simulink subsystem "robot_model_bus_7dof_ref_subsys"  (R2022b)
settings: Solver=VariableStepAuto  StartTime=0.0  StopTime=10.0  RelTol=1e-3
undefined symbols (not defined in the file): param_global
libraries: simulink x1
settings Model: Creator=emu  LastModifiedBy=emu
settings OptimizationCC: ReuseModelBlockBuffer=on

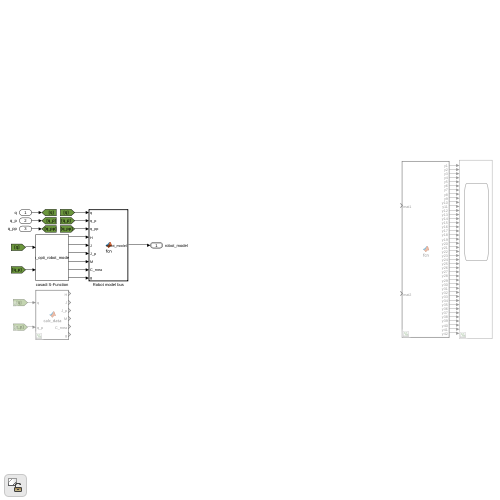
[thumbnail: Simulink's stored preview of the top-level diagram]
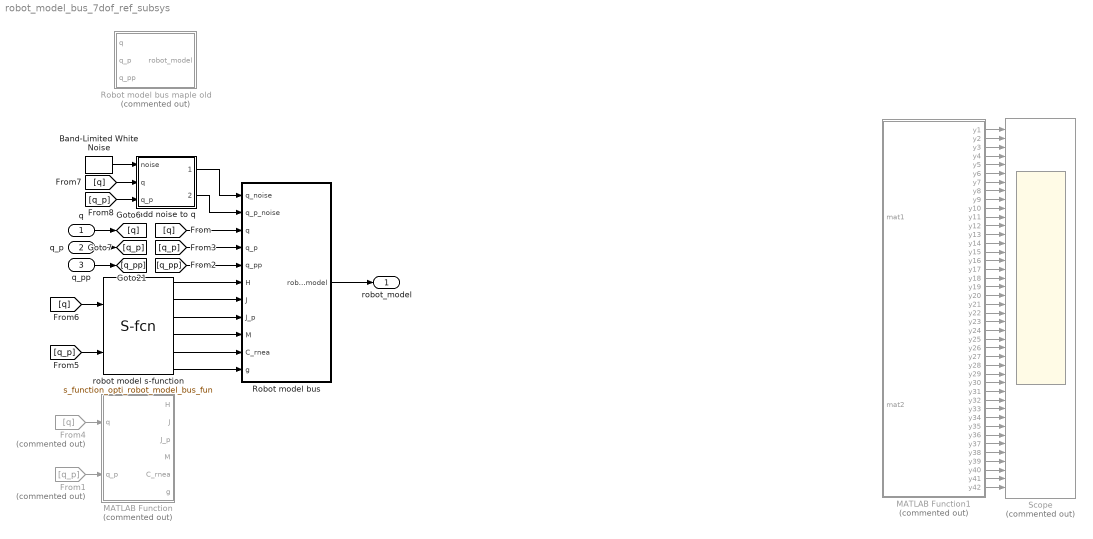
== system robot_model_bus_7dof_ref_subsys ==
  q : Inport
  q_p : Inport  Port=2
  q_pp : Inport  Port=3
  Band-Limited White Noise : simulink/Sources/Band-Limited White Noise  Cov=[1e-6]  Ts=param_global.Ta  seed=[23341]
  From1 : From  Commented=on  GotoTag=q_p
  From4 : From  Commented=on  GotoTag=q
  MATLAB Function : MATLAB Function  Commented=on  TreatAsAtomicUnit=on
  MATLAB Function1 : MATLAB Function  Commented=on  TreatAsAtomicUnit=on
  Robot model bus : MATLAB Function  TreatAsAtomicUnit=on
  Robot model bus maple old : MATLAB Function  Commented=on  TreatAsAtomicUnit=on
  Scope : Scope  Commented=on  NumInputPorts=42
  add noise to q : MATLAB Function  TreatAsAtomicUnit=on
  robot model s-function : S-Function  FunctionName=s_function_opti_robot_model_bus_fun  SFunctionModules='robot_model_bus_fun'  SFunctionDeploymentMode=off  EnableBusSupport=off
  robot_model : Outport  OutDataTypeStr=Bus: robot_model
  wires:
  Robot model bus/1(robot_model) -> robot_model/1
  robot model s-function/3 -> Robot model bus/8(J_p)
  robot model s-function/4 -> Robot model bus/9(M)
  robot model s-function/6 -> Robot model bus/11(g)
  q_pp/1 -> [q_pp]
  q_p/1 -> [q_p]
  q/1 -> [q]
  [q] -> Robot model bus/3(q)
  [q_p] -> Robot model bus/4(q_p)
  [q_pp] -> Robot model bus/5(q_pp)
  From4/1 -> MATLAB Function/1(q)
  From1/1 -> MATLAB Function/2(q_p)
  [q_p] -> robot model s-function/2
  [q] -> robot model s-function/1
  robot model s-function/5 -> Robot model bus/10(C_rnea)
  robot model s-function/1 -> Robot model bus/6(H)
  robot model s-function/2 -> Robot model bus/7(J)
  MATLAB Function1/1(y1) -> Scope/1
  MATLAB Function1/2(y2) -> Scope/2
  MATLAB Function1/3(y3) -> Scope/3
  MATLAB Function1/4(y4) -> Scope/4
  MATLAB Function1/5(y5) -> Scope/5
  MATLAB Function1/6(y6) -> Scope/6
  MATLAB Function1/7(y7) -> Scope/7
  MATLAB Function1/8(y8) -> Scope/8
  MATLAB Function1/9(y9) -> Scope/9
  MATLAB Function1/10(y10) -> Scope/10
  MATLAB Function1/11(y11) -> Scope/11
  MATLAB Function1/12(y12) -> Scope/12
  MATLAB Function1/13(y13) -> Scope/13
  MATLAB Function1/14(y14) -> Scope/14
  MATLAB Function1/15(y15) -> Scope/15
  MATLAB Function1/16(y16) -> Scope/16
  MATLAB Function1/17(y17) -> Scope/17
  MATLAB Function1/18(y18) -> Scope/18
  MATLAB Function1/19(y19) -> Scope/19
  MATLAB Function1/20(y20) -> Scope/20
  MATLAB Function1/21(y21) -> Scope/21
  MATLAB Function1/22(y22) -> Scope/22
  MATLAB Function1/23(y23) -> Scope/23
  MATLAB Function1/24(y24) -> Scope/24
  MATLAB Function1/25(y25) -> Scope/25
  MATLAB Function1/26(y26) -> Scope/26
  MATLAB Function1/27(y27) -> Scope/27
  MATLAB Function1/28(y28) -> Scope/28
  MATLAB Function1/29(y29) -> Scope/29
  MATLAB Function1/30(y30) -> Scope/30
  MATLAB Function1/31(y31) -> Scope/31
  MATLAB Function1/32(y32) -> Scope/32
  MATLAB Function1/33(y33) -> Scope/33
  MATLAB Function1/34(y34) -> Scope/34
  MATLAB Function1/35(y35) -> Scope/35
  MATLAB Function1/36(y36) -> Scope/36
  MATLAB Function1/37(y37) -> Scope/37
  MATLAB Function1/38(y38) -> Scope/38
  MATLAB Function1/39(y39) -> Scope/39
  MATLAB Function1/40(y40) -> Scope/40
  MATLAB Function1/41(y41) -> Scope/41
  MATLAB Function1/42(y42) -> Scope/42
  Band-Limited White Noise/1 -> add noise to q/1(noise)
  [q] -> add noise to q/2(q)
  [q_p] -> add noise to q/3(q_p)
  add noise to q/2(q_p_noise) -> Robot model bus/2(q_p_noise)
  add noise to q/1(q_noise) -> Robot model bus/1(q_noise)

== matlab function robot_model_bus_7dof_ref_subsys/Robot model bus maple old ==
  settings: updateMethod=DISCRETE  sampleTime=param_global.Ta
  data: q input; q_p input; q_pp input; robot_model output Bus: robot_model; param_robot parameter
function robot_model = fcn(q, q_p, q_pp, param_robot)
% Parameters
robot_model=struct();
robot_model.q=q;                    % generalized coordinates
robot_model.q_p=q_p;                % time derivative of generalized coordinates
robot_model.q_pp=q_pp;
robot_model.H=hom_transform_endeffector(q, param_robot);            % homogenous transformation to end-effector
robot_model.J=geo_jacobian_endeffector(q,param_robot);              % geometric jacobian to end-effector
robot_model.J_p=geo_jacobian_endeffector_p(q, q_p,param_robot);     % time derivative of geometric jacobian to end-effector
robot_model.M=inertia_matrix(q,param_robot);                        % inertia matrix
robot_model.C=coriolis_matrix(q, q_p,param_robot);                  % coriolis matrix
robot_model.g=gravitational_forces(q,param_robot);                  % gravitational forces
end

== matlab function robot_model_bus_7dof_ref_subsys/add noise to q ==
  data: noise input; q_noise output; q input; q_p input; q_p_noise output; param_global parameter
function [q_noise, q_p_noise] = fcn(noise, q, q_p, param_global)

q_noise = q + noise;
q_p_noise = q_p + param_global.Ta*noise;

== matlab function robot_model_bus_7dof_ref_subsys/Robot model bus ==
  settings: updateMethod=DISCRETE  sampleTime=param_global.Ta
  data: q_noise input; q_p_noise input; q input; q_p input; q_pp input; H input; J input; J_p input; M input; C_rnea input; g input; robot_model output Bus: robot_model
function robot_model = fcn(q_noise, q_p_noise, q, q_p, q_pp, H, J, J_p, M, C_rnea, g)
% Parameters
robot_model=struct();
robot_model.q_noise = q_noise;
robot_model.q_p_noise = q_p_noise;
robot_model.q=q;                    % generalized coordinates
robot_model.q_p=q_p;                % time derivative of generalized coordinates
robot_model.q_pp=q_pp;
robot_model.H=H;
robot_model.J=J;
robot_model.J_p=J_p;
robot_model.M=M;
robot_model.C_rnea=C_rnea; % C_rnea(q, q_p) = C(q, q_p)q_p + g(q) = n(q, q_p)
robot_model.g=g;
end

== matlab function robot_model_bus_7dof_ref_subsys/MATLAB Function ==
  data: q input; H output; q_p input; J output; J_p output; M output; C_rnea output; g output; param_robot parameter
function [H, J, J_p, M, C_rnea, g] = calc_data(q, q_p, param_robot)

H=hom_transform_endeffector(q, param_robot);            % homogenous transformation to end-effector
J=geo_jacobian_endeffector(q,param_robot);              % geometric jacobian to end-effector
J_p=geo_jacobian_endeffector_p(q, q_p,param_robot);     % time derivative of geometric jacobian to end-effector
M=inertia_matrix(q,param_robot);                        % inertia matrix
g=gravitational_forces(q,param_robot);                  % gravitational forces
C_rnea=coriolis_matrix(q, q_p,param_robot)*q_p + g;     % coriolis matrix

== matlab function robot_model_bus_7dof_ref_subsys/MATLAB Function1 ==
  data: mat1 input; y1 output Bus: test_bus; mat2 input; y2 output Bus: test_bus; y3 output Bus: test_bus; y4 output Bus: test_bus; y5 output Bus: test_bus; y6 output Bus: test_bus; y7 output Bus: test_bus; y8 output Bus: test_bus; y9 output Bus: test_bus; y10 output Bus: test_bus; y11 output Bus: test_bus; y12 output Bus: test_bus; y13 output Bus: test_bus; y14 output Bus: test_bus; y15 output Bus: test_bus; y16 output Bus: test_bus; y17 output Bus: test_bus; y18 output Bus: test_bus; y19 output Bus: test_bus; y20 output Bus: test_bus; y21 output Bus: test_bus; y22 output Bus: test_bus; y23 output Bus: test_bus; y24 output Bus: test_bus; y25 output Bus: test_bus; y26 output Bus: test_bus; y27 output Bus: test_bus; y28 output Bus: test_bus; y29 output Bus: test_bus; y30 output Bus: test_bus; y31 output Bus: test_bus; y32 output Bus: test_bus; y33 output Bus: test_bus; y34 output Bus: test_bus; y35 output Bus: test_bus; y36 output Bus: test_bus; y37 output Bus: test_bus; y38 output Bus: test_bus; y39 output Bus: test_bus; y40 output Bus: test_bus; y41 output Bus: test_bus; y42 output Bus: test_bus; init_bus_param parameter
function [y1, y2, y3, y4, y5, y6, y7, y8, y9, y10, y11, y12, y13, y14, y15, y16, y17, y18, y19, y20, y21, y22, y23, y24, y25, y26, y27, y28, y29, y30, y31, y32, y33, y34, y35, y36, y37, y38, y39, y40, y41, y42] = fcn(mat1, mat2, init_bus_param)
     
    y1 = init_bus_param.init_test_bus; y2 = init_bus_param.init_test_bus; y3 = init_bus_param.init_test_bus; y4 = init_bus_param.init_test_bus; y5 = init_bus_param.init_test_bus; y6 = init_bus_param.init_test_bus; y7 = init_bus_param.init_test_bus;
    y8 = init_bus_param.init_test_bus; y9 = init_bus_param.init_test_bus; y10 = init_bus_param.init_test_bus; y11 = init_bus_param.init_test_bus; y12 = init_bus_param.init_test_bus; y13 = init_bus_param.init_test_bus; y14 = init_bus_param.init_test_bus;
    y15 = init_bus_param.init_test_bus; y16 = init_bus_param.init_test_bus; y17 = init_bus_param.init_test_bus; y18 = init_bus_param.init_test_bus; y19 = init_bus_param.init_test_bus; y20 = init_bus_param.init_test_bus; y21 = init_bus_param.init_test_bus;
    y22 = init_bus_param.init_test_bus; y23 = init_bus_param.init_test_bus; y24 = init_bus_param.init_test_bus; y25 = init_bus_param.init_test_bus; y26 = init_bus_param.init_test_bus; y27 = init_bus_param.init_test_bus; y28 = init_bus_param.init_test_bus;
    y29 = init_bus_param.init_test_bus; y30 = init_bus_param.init_test_bus; y31 = init_bus_param.init_test_bus; y32 = init_bus_param.init_test_bus; y33 = init_bus_param.init_test_bus; y34 = init_bus_param.init_test_bus; y35 = init_bus_param.init_test_bus;
    y36 = init_bus_param.init_test_bus; y37 = init_bus_param.init_test_bus; y38 = init_bus_param.init_test_bus; y39 = init_bus_param.init_test_bus; y40 = init_bus_param.init_test_bus; y41 = init_bus_param.init_test_bus; y42 = init_bus_param.init_test_bus;
    

% Assign each struct to the corresponding output variable
    y1.mat_fun = mat1(1, 1); y1.pyt_fun = mat2(1, 1);
    y2.mat_fun = mat1(1, 2); y2.pyt_fun = mat2(1, 2);
    y3.mat_fun = mat1(1, 3); y3.pyt_fun = mat2(1, 3);
    y4.mat_fun = mat1(1, 4); y4.pyt_fun = mat2(1, 4);
    y5.mat_fun = mat1(1, 5); y5.pyt_fun = mat2(1, 5);
    y6.mat_fun = mat1(1, 6); y6.pyt_fun = mat2(1, 6);
    y7.mat_fun = mat1(1, 7); y7.pyt_fun = mat2(1, 7);
    y8.mat_fun = mat1(2, 1); y8.pyt_fun = mat2(2, 1);
    y9.mat_fun = mat1(2, 2); y9.pyt_fun = mat2(2, 2);
    y10.mat_fun = mat1(2, 3); y10.pyt_fun = mat2(2, 3);
    y11.mat_fun = mat1(2, 4); y11.pyt_fun = mat2(2, 4);
    y12.mat_fun = mat1(2, 5); y12.pyt_fun = mat2(2, 5);
    y13.mat_fun = mat1(2, 6); y13.pyt_fun = mat2(2, 6);
    y14.mat_fun = mat1(2, 7); y14.pyt_fun = mat2(2, 7);
    y15.mat_fun = mat1(3, 1); y15.pyt_fun = mat2(3, 1);
    y16.mat_fun = mat1(3, 2); y16.pyt_fun = mat2(3, 2);
    y17.mat_fun = mat1(3, 3); y17.pyt_fun = mat2(3, 3);
    y18.mat_fun = mat1(3, 4); y18.pyt_fun = mat2(3, 4);
    y19.mat_fun = mat1(3, 5); y19.pyt_fun = mat2(3, 5);
    y20.mat_fun = mat1(3, 6); y20.pyt_fun = mat2(3, 6);
    y21.mat_fun = mat1(3, 7); y21.pyt_fun = mat2(3, 7);
    y22.mat_fun = mat1(4, 1); y22.pyt_fun = mat2(4, 1);
    y23.mat_fun = mat1(4, 2); y23.pyt_fun = mat2(4, 2);
    y24.mat_fun = mat1(4, 3); y24.pyt_fun = mat2(4, 3);
    y25.mat_fun = mat1(4, 4); y25.pyt_fun = mat2(4, 4);
    y26.mat_fun = mat1(4, 5); y26.pyt_fun = mat2(4, 5);
    y27.mat_fun = mat1(4, 6); y27.pyt_fun = mat2(4, 6);
    y28.mat_fun = mat1(4, 7); y28.pyt_fun = mat2(4, 7);
    y29.mat_fun = mat1(5, 1); y29.pyt_fun = mat2(5, 1);
    y30.mat_fun = mat1(5, 2); y30.pyt_fun = mat2(5, 2);
    y31.mat_fun = mat1(5, 3); y31.pyt_fun = mat2(5, 3);
    y32.mat_fun = mat1(5, 4); y32.pyt_fun = mat2(5, 4);
    y33.mat_fun = mat1(5, 5); y33.pyt_fun = mat2(5, 5);
    y34.mat_fun = mat1(5, 6); y34.pyt_fun = mat2(5, 6);
    y35.mat_fun = mat1(5, 7); y35.pyt_fun = mat2(5, 7);
    y36.mat_fun = mat1(6, 1); y36.pyt_fun = mat2(6, 1);
    y37.mat_fun = mat1(6, 2); y37.pyt_fun = mat2(6, 2);
    y38.mat_fun = mat1(6, 3); y38.pyt_fun = mat2(6, 3);
    y39.mat_fun = mat1(6, 4); y39.pyt_fun = mat2(6, 4);
    y40.mat_fun = mat1(6, 5); y40.pyt_fun = mat2(6, 5);
    y41.mat_fun = mat1(6, 6); y41.pyt_fun = mat2(6, 6);
    y42.mat_fun = mat1(6, 7); y42.pyt_fun = mat2(6, 7);
end
